simulink model "QuaternionPDRotate"  (R2021b)
settings: Solver=VariableStepAuto  StartTime=0.0  StopTime=20  RelTol=1e-3
libraries: aerolibutil x6, simulink x3, Contact_Forces_Lib x2, sharedtransform x2, sharedutil x1, cstblocks x1
settings Model: Creator=thinkpad  LastModifiedBy=thinkpad

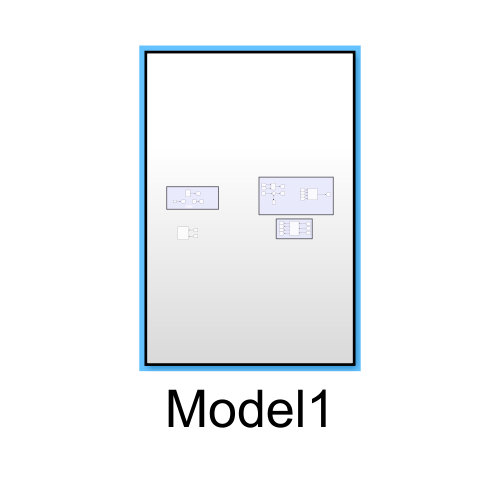
[thumbnail: Simulink's stored preview of the top-level diagram]
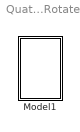
== system QuaternionPDRotate ==
  Model1 : Subsystem

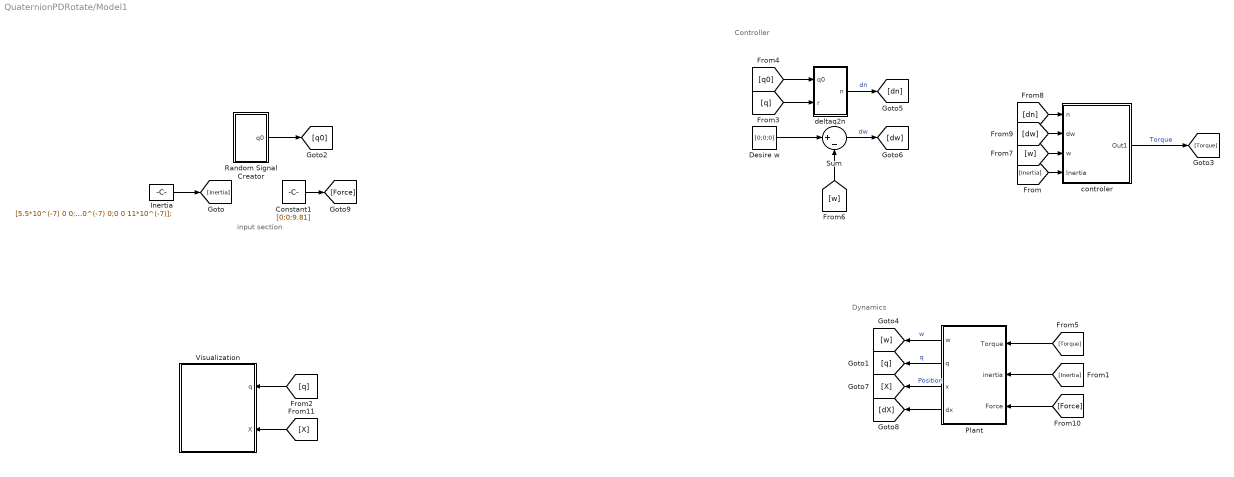
== system QuaternionPDRotate/Model1 ==
  note: input section
  note: Controller
  note: Dynamics
  Constant1 : Constant  Value=[0;0;9.81]
  Desire w : Constant  Value=[0;0;0]
  Inertia : Constant  Value=[5.5*10^(-7) 0 0;0 5.5*10^(-7) 0;0 0 11*10^(-7)];
  Plant : Subsystem
  Random Signal Creator : Subsystem
  Sum : Sum  Inputs=|+-
  Visualization : Subsystem
  controler : Subsystem
  deltaq2n : Subsystem
  wires:
  Plant/2(q) -> [q]  "q"
  Plant/4(dx) -> [dX]
  Inertia/1 -> [Inertia]
  [dw] -> controler/2(dw)
  Random Signal Creator/1(q0) -> [q0]
  [q0] -> deltaq2n/1(q0)
  [w] -> Sum/2
  Sum/1 -> [dw]  "dw"
  [w] -> controler/3(w)
  Plant/3(x) -> [X]  "Position"
  [q] -> deltaq2n/2(r)
  Constant1/1 -> [Force]
  Plant/1(w) -> [w]  "w"
  [dn] -> controler/1(n)
  [Inertia] -> controler/4(Inertia)
  deltaq2n/1(n) -> [dn]  "dn"
  [q] -> Visualization/1(q)
  [Force] -> Plant/3(Force)
  controler/1(Out1) -> [Torque]  "Torque"
  [Inertia] -> Plant/2(inertia)
  [Torque] -> Plant/1(Torque)
  Desire w/1 -> Sum/1
  [X] -> Visualization/2(X)

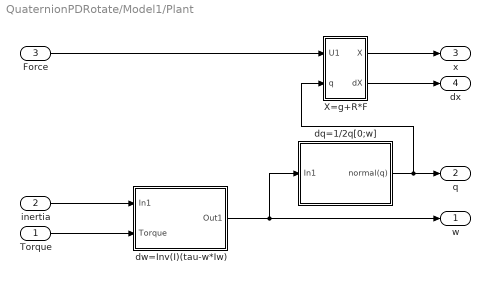
== system QuaternionPDRotate/Model1/Plant ==
  Torque : Inport  PortDimensions=3
  inertia : Inport  Port=2
  Force : Inport  Port=3
  X=g+R*F : Subsystem
  dq=1/2q[0;w] : Subsystem
  dw=Inv(I)(tau-w*Iw) : Subsystem
  w : Outport
  q : Outport  Port=2
  x : Outport  Port=3
  dx : Outport  Port=4
  wires:
  dw=Inv(I)(tau-w*Iw)/1(Out1) -> w/1, dq=1/2q[0;w]/1(In1)
  inertia/1 -> dw=Inv(I)(tau-w*Iw)/1(In1)
  Torque/1 -> dw=Inv(I)(tau-w*Iw)/2(Torque)
  dq=1/2q[0;w]/1(normal(q)) -> X=g+R*F/2(q), q/1
  Force/1 -> X=g+R*F/1(U1)
  X=g+R*F/1(X) -> x/1
  X=g+R*F/2(dX) -> dx/1

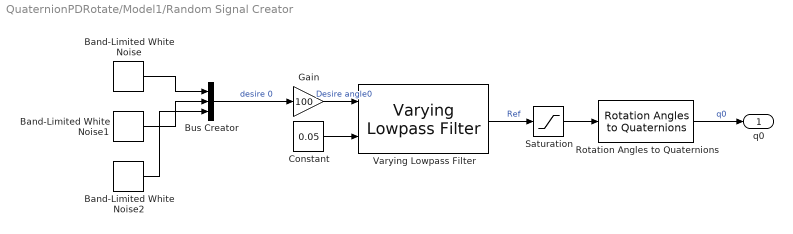
== system QuaternionPDRotate/Model1/Random Signal Creator ==
  Band-Limited White Noise : simulink/Sources/Band-Limited White Noise  Cov=[0.005]  Ts=1e-3  seed=[23341]  VectorParams1D=off
  Band-Limited White Noise1 : simulink/Sources/Band-Limited White Noise  Cov=[0.005]  Ts=1e-3  seed=[23342]  VectorParams1D=off
  Band-Limited White Noise2 : simulink/Sources/Band-Limited White Noise  Cov=[0.005]  Ts=1e-3  seed=[23343]  VectorParams1D=off
  Bus Creator : BusCreator  Inputs=3
  Constant : Constant  Value=0.05
  Gain : Gain  Gain=100
  Rotation Angles to Quaternions : sharedtransform/Rotation Angles to Quaternions  rotationOrder=ZYX  aMode=aMode
      settings: SourceProductBaseCode=AE,PW,DR,MT,UV,VE
  Saturation : Saturate  UpperLimit=[pi;pi/2;pi/2]  LowerLimit=[-pi;-pi/2;-pi/2]
  Varying Lowpass Filter : cstblocks/Linear Parameter Varying/Varying Lowpass Filter  N=1
  q0 : Outport
  wires:
  Band-Limited White Noise1/1 -> Bus Creator/2
  Band-Limited White Noise2/1 -> Bus Creator/3
  Gain/1 -> Varying Lowpass Filter/1  "Desire angle0"
  Band-Limited White Noise/1 -> Bus Creator/1
  Varying Lowpass Filter/1 -> Saturation/1  "Ref"
  Bus Creator/1 -> Gain/1  "desire 0"
  Constant/1 -> Varying Lowpass Filter/2
  Saturation/1 -> Rotation Angles to Quaternions/1
  Rotation Angles to Quaternions/1 -> q0/1  "q0"

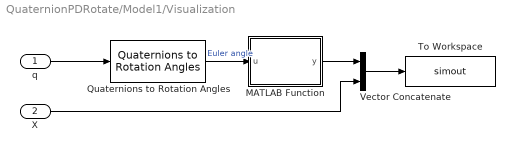
== system QuaternionPDRotate/Model1/Visualization ==
  q : Inport
  X : Inport  Port=2
  MATLAB Function : MATLAB Function  TreatAsAtomicUnit=on
  Quaternions to Rotation Angles : sharedtransform/Quaternions to Rotation Angles  rotationOrder=ZYX  aMode=aMode
      settings: SourceProductBaseCode=AE,PW,DR,MT,UV,VE
  To Workspace : ToWorkspace  VariableName=simout  SampleTime=-1
      settings: Save2DSignal=2-D array (concatenate along first dimension)
  Vector Concatenate : Concatenate
  wires:
  q/1 -> Quaternions to Rotation Angles/1
  Quaternions to Rotation Angles/1 -> MATLAB Function/1(u)  "Euler angle"
  MATLAB Function/1(y) -> Vector Concatenate/1
  Vector Concatenate/1 -> To Workspace/1
  X/1 -> Vector Concatenate/2

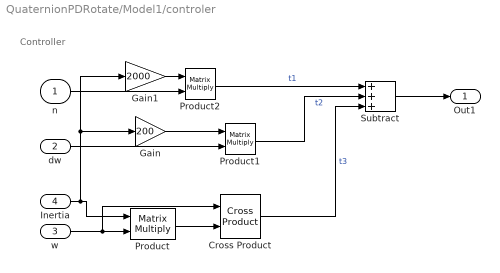
== system QuaternionPDRotate/Model1/controler ==
  note: Controller
  n : Inport
  dw : Inport  Port=2  PortDimensions=3
  w : Inport  Port=3
  Inertia : Inport  Port=4
  Cross Product : Contact_Forces_Lib/Math/Cross Product  SystemSampleTime=-1  VariantActivationTime=update diagram  Latency=0  AutoFrameSizeCalculation=off
      settings: SourceProductName=Simscape Multibody Contact Forces Library
  Gain : Gain  Gain=200
  Gain1 : Gain  Gain=2000
  Product : Product  Multiplication=Matrix(*)
  Product1 : Product  Multiplication=Matrix(*)
  Product2 : Product  Multiplication=Matrix(*)
  Subtract : Sum  Inputs=+++
  Out1 : Outport
  wires:
  Product1/1 -> Subtract/2  "t2"
  Product/1 -> Cross Product/2
  w/1 -> Cross Product/1, Product/2
  Subtract/1 -> Out1/1
  Inertia/1 -> Gain1/1, Gain/1, Product/1
  Product2/1 -> Subtract/1  "t1"
  Gain1/1 -> Product2/1
  n/1 -> Product2/2
  Gain/1 -> Product1/1
  dw/1 -> Product1/2
  Cross Product/1 -> Subtract/3  "t3"

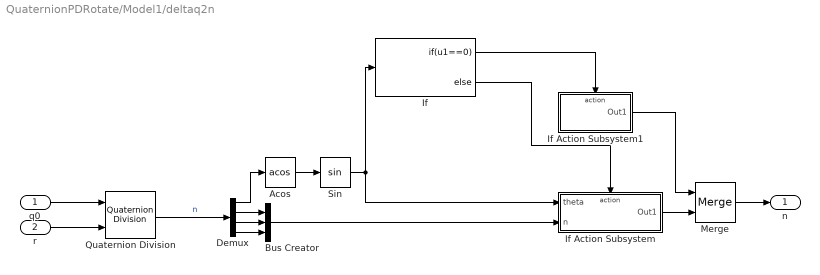
== system QuaternionPDRotate/Model1/deltaq2n ==
  q0 : Inport
  r : Inport  Port=2
  Acos : Trigonometry  Operator=acos
  Bus Creator : BusCreator  Inputs=3
  Demux : Demux
  If : If  IfExpression=u1==0
  If Action Subsystem : Subsystem  TreatAsAtomicUnit=on
  If Action Subsystem1 : Subsystem  TreatAsAtomicUnit=on
  Merge : Merge
  Quaternion Division : aerolibutil/Quaternion Division
      settings: SourceProductBaseCode=AE
  Sin : Trigonometry
  n : Outport
  wires:
  Demux/4 -> Bus Creator/3
  Bus Creator/1 -> If Action Subsystem/2(n)
  Quaternion Division/1 -> Demux/1  "n"
  Sin/1 -> If Action Subsystem/1(theta), If/1
  Acos/1 -> Sin/1
  Demux/2 -> Bus Creator/1
  Demux/3 -> Bus Creator/2
  Demux/1 -> Acos/1
  r/1 -> Quaternion Division/2
  q0/1 -> Quaternion Division/1
  If Action Subsystem/1(Out1) -> Merge/2
  Merge/1 -> n/1
  If/2 -> If Action Subsystem/Action
  If/1 -> If Action Subsystem1/Action
  If Action Subsystem1/1(Out1) -> Merge/1

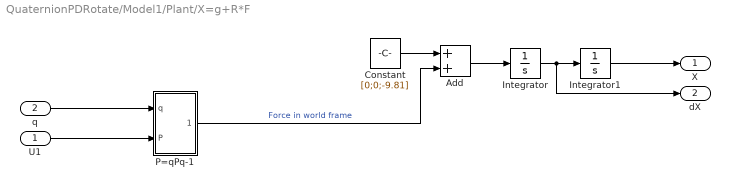
== system QuaternionPDRotate/Model1/Plant/X=g+R*F ==
  U1 : Inport
  q : Inport  Port=2
  Add : Sum
  Constant : Constant  Value=[0;0;-9.81]
  Integrator : Integrator  InitialCondition=[0;0;0]
  Integrator1 : Integrator  InitialCondition=[0;0;0]
  P=qPq-1 : Subsystem
  X : Outport
  dX : Outport  Port=2
  wires:
  Integrator/1 -> dX/1, Integrator1/1
  Add/1 -> Integrator/1
  Constant/1 -> Add/1
  Integrator1/1 -> X/1
  q/1 -> P=qPq-1/1(q)
  U1/1 -> P=qPq-1/2(P)
  P=qPq-1/1(Out1) -> Add/2  "Force in world frame"

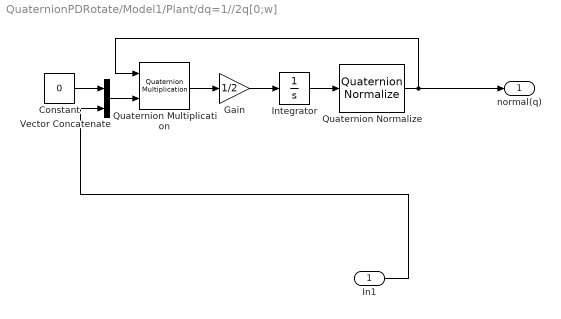
== system QuaternionPDRotate/Model1/Plant/dq=1//2q[0;w] ==
  In1 : Inport
  Constant : Constant  Value=0
  Gain : Gain  Gain=1/2
  Integrator : Integrator  InitialCondition=[1;0;0;0]
  Quaternion Multiplication : aerolibutil/Quaternion Multiplication
  Quaternion Normalize : sharedutil/Quaternion Normalize  aMode=aMode
      settings: SourceProductBaseCode=AE,PW,DR,MT,UV,VE
  Vector Concatenate : Concatenate
  normal(q) : Outport
  wires:
  Quaternion Normalize/1 -> normal(q)/1, Quaternion Multiplication/1
  Integrator/1 -> Quaternion Normalize/1
  In1/1 -> Vector Concatenate/2
  Constant/1 -> Vector Concatenate/1
  Vector Concatenate/1 -> Quaternion Multiplication/2
  Quaternion Multiplication/1 -> Gain/1
  Gain/1 -> Integrator/1

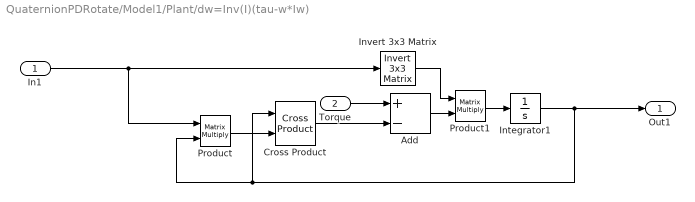
== system QuaternionPDRotate/Model1/Plant/dw=Inv(I)(tau-w*Iw) ==
  In1 : Inport
  Torque : Inport  Port=2  PortDimensions=3
  Add : Sum  Inputs=+-
  Cross Product : Contact_Forces_Lib/Math/Cross Product  SystemSampleTime=-1  VariantActivationTime=update diagram  Latency=0  AutoFrameSizeCalculation=off
      settings: SourceProductName=Simscape Multibody Contact Forces Library
  Integrator1 : Integrator  InitialCondition=[0;0;0]
  Invert 3x3 Matrix : aerolibutil/Invert  3x3 Matrix
  Product : Product  Multiplication=Matrix(*)
  Product1 : Product  Multiplication=Matrix(*)
  Out1 : Outport
  wires:
  Product1/1 -> Integrator1/1
  Cross Product/1 -> Add/2
  Integrator1/1 -> Out1/1, Cross Product/1, Product/2
  Add/1 -> Product1/2
  In1/1 -> Invert 3x3 Matrix/1, Product/1
  Product/1 -> Cross Product/2
  Torque/1 -> Add/1
  Invert 3x3 Matrix/1 -> Product1/1

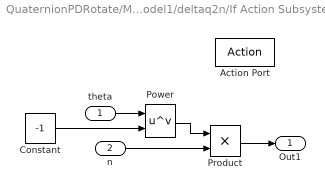
== system QuaternionPDRotate/Model1/deltaq2n/If Action Subsystem ==
  theta : Inport
  n : Inport  Port=2
  Action Port : ActionPort  ActionPortLabel=else
  Constant : Constant  Value=-1
  Power : Math  Operator=pow  SaturateOnIntegerOverflow=on
  Product : Product
  Out1 : Outport
  wires:
  Product/1 -> Out1/1
  theta/1 -> Power/1
  n/1 -> Product/2
  Power/1 -> Product/1
  Constant/1 -> Power/2

== system QuaternionPDRotate/Model1/deltaq2n/If Action Subsystem1 ==
  Action Port : ActionPort  ActionPortLabel=if(u1==0)
  Constant : Constant  Value=[0;0;0]
  Out1 : Outport
  wires:
  Constant/1 -> Out1/1

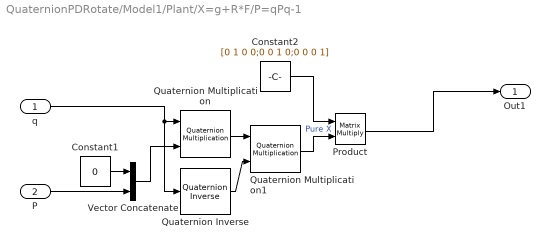
== system QuaternionPDRotate/Model1/Plant/X=g+R*F/P=qPq-1 ==
  q : Inport
  P : Inport  Port=2
  Constant1 : Constant  Value=0
  Constant2 : Constant  Value=[0 1 0 0;0 0 1 0;0 0 0 1]
  Product : Product  Multiplication=Matrix(*)
  Quaternion Inverse : aerolibutil/Quaternion Inverse
  Quaternion Multiplication : aerolibutil/Quaternion Multiplication
  Quaternion Multiplication1 : aerolibutil/Quaternion Multiplication
  Vector Concatenate : Concatenate
  Out1 : Outport
  wires:
  Quaternion Multiplication1/1 -> Product/2  "Pure X"
  q/1 -> Quaternion Inverse/1, Quaternion Multiplication/1
  Constant2/1 -> Product/1
  Vector Concatenate/1 -> Quaternion Multiplication/2
  Constant1/1 -> Vector Concatenate/1
  Quaternion Inverse/1 -> Quaternion Multiplication1/2
  Product/1 -> Out1/1
  Quaternion Multiplication/1 -> Quaternion Multiplication1/1
  P/1 -> Vector Concatenate/2

== matlab function QuaternionPDRotate/Model1/Visualization/MATLAB Function ==
  data: u input; y output
function y = fcn(u)
for i=1:3
    if u(i)> pi
        u(i)=u(i)-2*pi;
    end
end
y = u.';
